simulink model "calibration_R2022b"  (R2022b)
settings: Solver=VariableStepAuto  StartTime=0.0  StopTime=1  RelTol=1e-3
libraries: robotgazebolib x2, dspvision x1, visionsinks x1
settings Model: LastModifiedBy=22546723@sun.ac.za
settings OptimizationCC: ReuseModelBlockBuffer=on

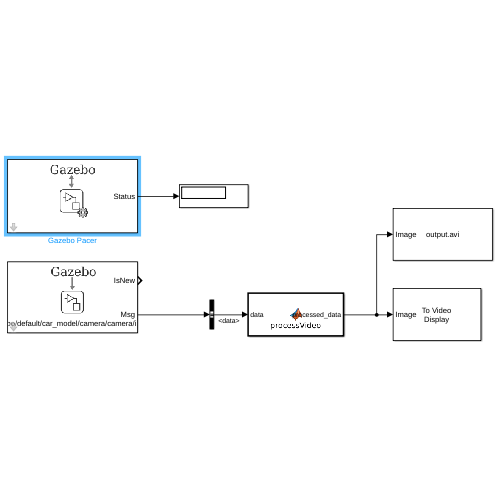
[thumbnail: Simulink's stored preview of the top-level diagram]
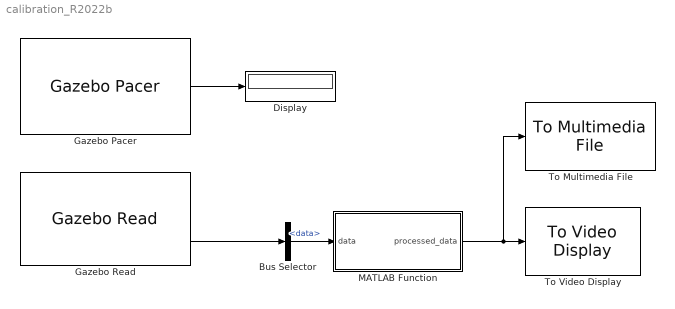
== system calibration_R2022b ==
  Bus Selector : BusSelector  OutputSignals=data
  Display : Display
  Gazebo Pacer : robotgazebolib/Gazebo Pacer  ResetBehavior=Reset Gazebo simulation time  SampleTime=0.001
  Gazebo Read : robotgazebolib/Gazebo Read  topicSource=From Gazebo  topic=/gazebo/default/car_model/camera/camera/image  messageType=gazebo_msgs/Image  sampleTime=0.001  fixedAxisBusStatus=off  jointAxisCount=2
  MATLAB Function : MATLAB Function  TreatAsAtomicUnit=on
  To Multimedia File : dspvision/To Multimedia File  outputFilename=output.avi  streamSelection=Video only  videoCompressor=None (uncompressed)  audioCompressor=None (uncompressed)  imagePorts=One multidimensional signal  fileType=AVI  audioDatatype=Determine from input data type  fourcc=RGB  videoQuality=75  mj2000CompFactor=10
      settings: LibrarySourceBlock=visionsinks/To Multimedia File
  To Video Display : visionsinks/To Video Display  windowSizeMode=Normal  openAtMdlStart=on  fullScreen=off  videoWindowX=536805376  videoWindowY=536805376  saveWindowSize=off  videoWindowWidth=2147483647  videoWindowHeight=2147483647  inputColorFormat=RGB  inputType=Obsolete  imagePorts=One multidimensional signal  OutputDevice=On-screen video monitor  dataOrg=Column-major  isWindowOpen=off
  wires:
  Gazebo Read/2 -> Bus Selector/1
  MATLAB Function/1(processed_data) -> To Multimedia File/1, To Video Display/1
  Bus Selector/1 -> MATLAB Function/1(data)  "<data>"
  Gazebo Pacer/1 -> Display/1

== matlab function calibration_R2022b/MATLAB Function ==
  data: data input; processed_data output
function processed_data=processVideo(data)
% the camera sends a 1200*600*3 data signal. Simulink receives it as a 1-D
% array

width = 1200;
height = 600;
z = 3;

processed_data = zeros(height, width, z, 'uint8');

if ~isempty(data) && ~isscalar(data)

    indexBase = (1:z:width*height*z)';
    index = zeros(numel(indexBase), z);

    for i=1:z
        index(:, i) = indexBase + i - 1;
    end

    temp = reshape(data(index), width, height, z);
    processed_data = permute(temp, [2 1 3]);

end
